simulink model "feedback_loop_Xi_Turb_var_char_2"  (Simulink 7.9)
settings: Solver=ode45  StartTime=0.0  StopTime=2000  RelTol=1e-3
settings Model: Creator=kr2112  LastModifiedBy=kr2112
settings DebuggingCC: MaxConsecutiveZCsMsg=warning

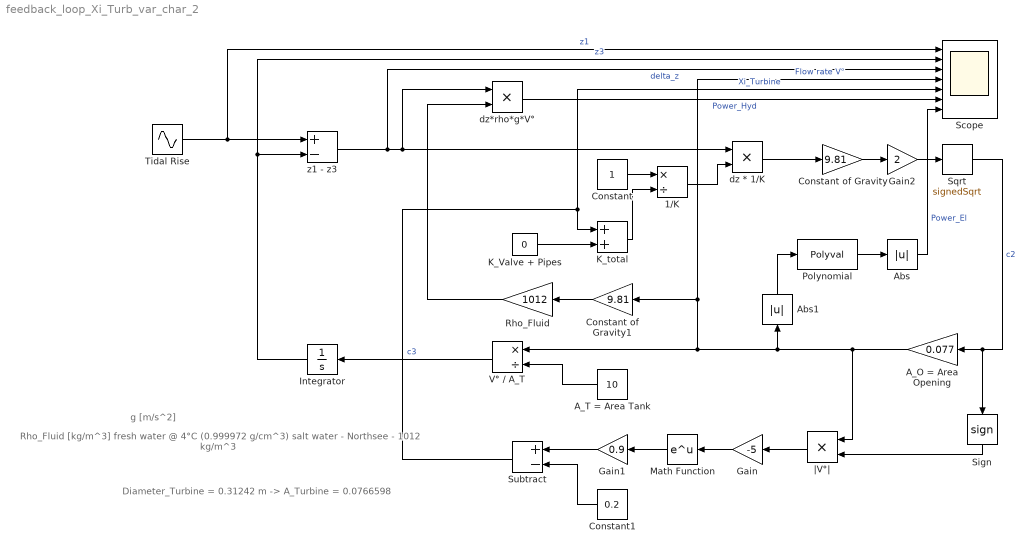
== system feedback_loop_Xi_Turb_var_char_2 ==
  note: Rho_Fluid [kg/m^3]
      | fresh water @ 4°C (0.999972 g/cm^3)
      | salt water - Northsee - 1012 kg/m^3
  note: g [m/s^2]
  note: Diameter_Turbine = 0.31242 m -> A_Turbine = 0.0766598
  1/K : Product  Inputs=*/
  A_O = Area Opening : Gain  Gain=0.077
  A_T = Area Tank : Constant  Value=10
  Abs : Abs
  Abs1 : Abs
  Constant : Constant
  Constant of Gravity : Gain  Gain=9.81
  Constant of Gravity1 : Gain  Gain=9.81
  Constant1 : Constant  Value=0.2
  Gain : Gain  Gain=-5
  Gain1 : Gain  Gain=0.9
  Gain2 : Gain  Gain=2
  Integrator : Integrator
  K_Valve + Pipes : Constant  Value=0
  K_total : Sum
  Math Function : Math  SaturateOnIntegerOverflow=on
  Polynomial : Polyval  Coefs=[ +1.9891e+03, -2.0277e+03, +0.9206e+03,-0.0488e+03 ]
  Rho_Fluid : Gain  Gain=1012
  Scope : Scope  NumInputPorts=7
      settings: YMin=-5~-5~-5~-5~-5~-5~-5  YMax=5~5~5~5~5~5~5
  Sign : Signum
  Sqrt : Sqrt  Operator=signedSqrt  SaturateOnIntegerOverflow=on
  Subtract : Sum  Inputs=+-
  Tidal Rise : Sin  Amplitude=2  Frequency=0.0083  SampleTime=0
  V° / A_T : Product  Inputs=*/
  dz * 1/K : Product  RndMeth=Zero
  dz*rho*g*V° : Product  RndMeth=Zero
  z1 - z3 : Sum  Inputs=+-
  |V°| : Product  RndMeth=Zero
  wires:
  Sqrt/1 -> A_O = Area Opening/1, Sign/1  "c2"
  z1 - z3/1 -> Scope/3, dz*rho*g*V°/1, dz * 1/K/1  "delta_z"
  Tidal Rise/1 -> z1 - z3/1, Scope/1  "z1"
  Integrator/1 -> Scope/2, z1 - z3/2  "z3"
  Gain2/1 -> Sqrt/1
  A_T = Area Tank/1 -> V° / A_T/2
  V° / A_T/1 -> Integrator/1  "c3"
  dz*rho*g*V°/1 -> Scope/6  "Power_Hyd"
  Constant of Gravity1/1 -> Rho_Fluid/1
  Rho_Fluid/1 -> dz*rho*g*V°/2
  A_O = Area Opening/1 -> |V°|/1, Abs1/1, V° / A_T/1, Constant of Gravity1/1, Scope/4  "Flow rate V°"
  Constant of Gravity/1 -> Gain2/1
  K_total/1 -> 1/K/2
  Constant/1 -> 1/K/1
  K_Valve + Pipes/1 -> K_total/2
  dz * 1/K/1 -> Constant of Gravity/1
  1/K/1 -> dz * 1/K/2
  Sign/1 -> |V°|/2
  |V°|/1 -> Gain/1
  Gain/1 -> Math Function/1
  Math Function/1 -> Gain1/1
  Gain1/1 -> Subtract/1
  Constant1/1 -> Subtract/2
  Subtract/1 -> K_total/1, Scope/5  "Xi_Turbine"
  Polynomial/1 -> Abs/1
  Abs1/1 -> Polynomial/1
  Abs/1 -> Scope/7  "Power_El"
